simulink model "WDGTTCCalculation_Harness"  (R2024a)
settings: configuration reference "csMultiInstance" (kept outside this file)
settings Model: DataDictionary=DD_WDGTTCCalculation.sldd  Creator=The MathWorks, Inc.  LastModifiedBy=The MathWorks, Inc.
settings ConfigSetRef: SourceName=csMultiInstance

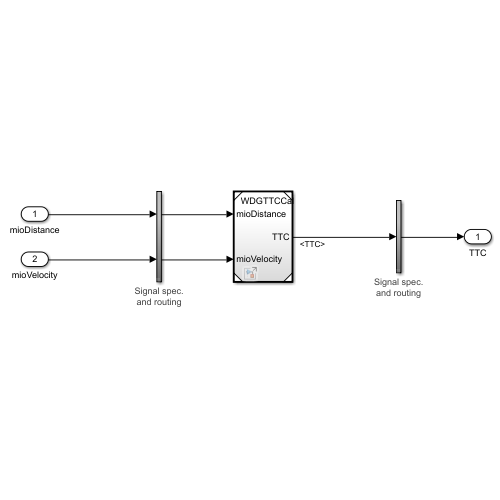
[thumbnail: Simulink's stored preview of the top-level diagram]
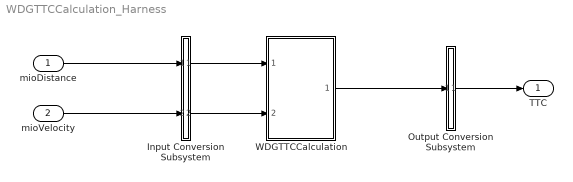
== system WDGTTCCalculation_Harness ==
  mioDistance : Inport  OutDataTypeStr=double  PortDimensions=[1]  SampleTime=0.1
  mioVelocity : Inport  Port=2  OutDataTypeStr=double  PortDimensions=[1]  SampleTime=0.1
  Input Conversion Subsystem : Subsystem  Tag=__SLT_ICS__  Description=|
      | Signal spec.
      | and routing
      settings: AttributesFormatString=%<Description>
  Output Conversion Subsystem : Subsystem  Tag=__SLT_OCS__  Description=|
      | Signal spec.
      | and routing
      settings: AttributesFormatString=%<Description>
  WDGTTCCalculation : ModelReference  ModelNameDialog=WDGTTCCalculation  SimulationMode=Normal  ModelReferenceVersion=7.0
  TTC : Outport
  wires:
  mioDistance/1 -> Input Conversion Subsystem/1(Inport_1)
  mioVelocity/1 -> Input Conversion Subsystem/2(Inport_2)
  Output Conversion Subsystem/1(Outport_1) -> TTC/1
  Input Conversion Subsystem/1(Outport_1) -> WDGTTCCalculation/1
  Input Conversion Subsystem/2(Outport_2) -> WDGTTCCalculation/2
  WDGTTCCalculation/1 -> Output Conversion Subsystem/1(Inport_1)

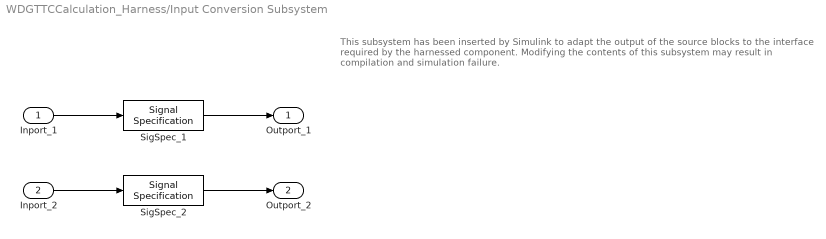
== system WDGTTCCalculation_Harness/Input Conversion Subsystem ==
  note: This subsystem has been inserted by Simulink to adapt the output of the source blocks to the interface required by the harnessed component.
      |  Modifying the contents of this subsystem may result in compilation and simulation failure.
  Inport_1 : Inport
  Inport_2 : Inport  Port=2
  SigSpec_1 : SignalSpecification  OutDataTypeStr=double  Unit=m  Dimensions=[1]  SampleTime=0.1
  SigSpec_2 : SignalSpecification  OutDataTypeStr=double  Unit=m/s  Dimensions=[1]  SampleTime=0.1
  Outport_1 : Outport
  Outport_2 : Outport  Port=2
  wires:
  SigSpec_1/1 -> Outport_1/1
  Inport_1/1 -> SigSpec_1/1
  SigSpec_2/1 -> Outport_2/1
  Inport_2/1 -> SigSpec_2/1

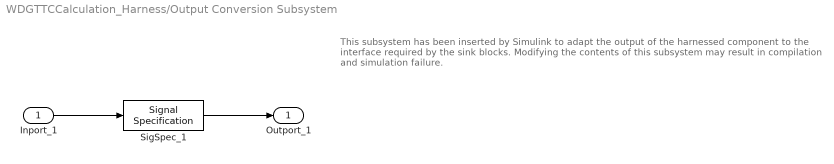
== system WDGTTCCalculation_Harness/Output Conversion Subsystem ==
  note: This subsystem has been inserted by Simulink to adapt the output of the harnessed component to the interface required by the sink blocks.
      |  Modifying the contents of this subsystem may result in compilation and simulation failure.
  Inport_1 : Inport
  SigSpec_1 : SignalSpecification  OutDataTypeStr=double  Unit=s  Dimensions=[1]  SampleTime=0.1
  Outport_1 : Outport
  wires:
  Inport_1/1 -> SigSpec_1/1
  SigSpec_1/1 -> Outport_1/1
